simulink model "Cardiovascular"  (Simulink 6.4)
settings: Solver=ode45  StartTime=0.0  StopTime=50  MaxStep=0.01  MinStep=0.0000000000001  RelTol=1e-1
values from neighbouring files (symbols this model uses):
  A = 20.9    [Gas_Exchange_IC.m]    (also in getPneumonia.m = (LF1-LF2)/(1-exp(Rresolve*(t2(end)-t2(1)))))
  B = 92.8    [Gas_Exchange_IC.m]    (also in getPneumonia.m = LungFunction(end)-A)
  C = 10570    [Gas_Exchange_IC.m]
  D = -5.251    [Gas_Exchange_IC.m]
  fcs_max = 47.78    [Cardiovascular_IC.m]    (also in Reflex_Ursino_IC.m)
  fcs_min = 2.52    [Cardiovascular_IC.m]    (also in Reflex_Ursino_IC.m)
  ftbs_min = 0.1    [Cardiovascular_IC.m]    (also in SA_Node_Ursino_IC.m)
  HP_basal = 0.58    [Cardiovascular_IC.m]    (also in SA_Node_Ursino_IC.m)
  k_cs = 11.758    [Cardiovascular_IC.m]    (also in Reflex_Ursino_IC.m)
  Pn = 90    [Cardiovascular_IC.m]    (also in Reflex_Ursino_IC.m)
undefined symbols (not defined in the file or in its folder): Cbp, Cbv, Cep, Cev, Chp, Chv, Cla, Cmp, Cmv, Cpa, Cpp, Cpv, Cra, Csa, Csp, Csv, CvbO2_n, CvhO2_n, CvmO2_n, Dx, ftas_min, Gas_sleep, GbO2, Gbs_sleep, GhO2, GmO2, Gpara_sleep, initx, k_cs_sleep, KElv, KErv, KhCO2, KmCO2, Kr_vc, KRlv, KRrv, ksys, Lpa, Lsa, Mb, Mhn, Mm, P0lv, P0rv, PaCO2_n, Pn_sleep, R_vc_0, Rbpn, Rbv, Rev, Rhpn, Rhv, Rla, Rmv, Rpa, Rpp, Rpv, Rra, Rsa, Rsv ... (+25)
(part 1 of 2)
settings Model: LastModifiedBy=cPhonix
settings SolverCC: InitialStep=0.0000000000001
settings DataIOCC: SignalLoggingName=sigsOut
settings OptimizationCC: BooleanDataType=off
settings DebuggingCC: SolverPrmCheckMsg=none  StrictBusMsg=None
settings HardwareCC: TargetUnknown=on

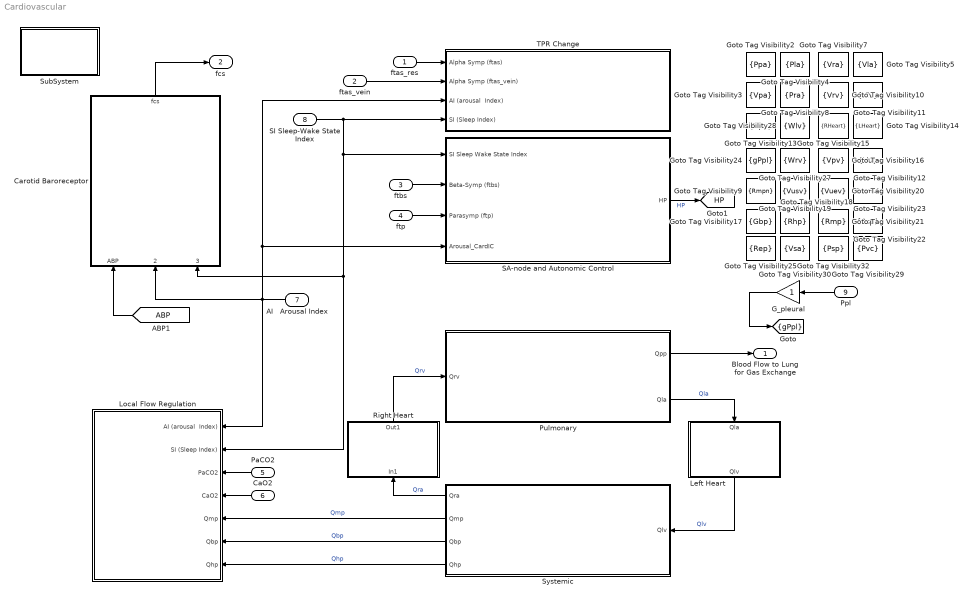
== system Cardiovascular ==
  ftas_res : Inport
  ftas_vein : Inport  Port=2
  ftbs : Inport  Port=3
  ftp : Inport  Port=4
  PaCO2 : Inport  Orientation=left  Port=5
  CaO2 : Inport  Orientation=left  Port=6
  AI   Arousal Index : Inport  Orientation=left  Port=7  DataType=double
  SI Sleep-Wake State Index : Inport  Port=8
  Ppl : Inport  Orientation=left  Port=9
  Carotid Baroreceptor : Subsystem  Orientation=up
      mask Display: disp('Carotid\n Baroreceptor')
  G_pleural : Gain  Orientation=left  SaturateOnIntegerOverflow=on
  Goto Tag Visibility10 : GotoTagVisibility  GotoTag=Vrv
  Goto Tag Visibility11 : GotoTagVisibility  GotoTag=Vlv
  Goto Tag Visibility12 : GotoTagVisibility  GotoTag=Vu
  Goto Tag Visibility13 : GotoTagVisibility  GotoTag=Vpp
  Goto Tag Visibility14 : GotoTagVisibility  GotoTag=LHeart
  Goto Tag Visibility15 : GotoTagVisibility  GotoTag=RHeart
  Goto Tag Visibility16 : GotoTagVisibility  GotoTag=Vpv
  Goto Tag Visibility17 : GotoTagVisibility  GotoTag=Gbp
  Goto Tag Visibility18 : GotoTagVisibility  GotoTag=Rhp
  Goto Tag Visibility19 : GotoTagVisibility  GotoTag=Vusv
  Goto Tag Visibility2 : GotoTagVisibility  GotoTag=Ppa
  Goto Tag Visibility20 : GotoTagVisibility  GotoTag=Vuev
  Goto Tag Visibility21 : GotoTagVisibility  GotoTag=Rmp
  Goto Tag Visibility22 : GotoTagVisibility  GotoTag=Rsp
  Goto Tag Visibility23 : GotoTagVisibility  GotoTag=Vumv
  Goto Tag Visibility24 : GotoTagVisibility  GotoTag=gPpl
  Goto Tag Visibility25 : GotoTagVisibility  GotoTag=Rep
  Goto Tag Visibility27 : GotoTagVisibility  GotoTag=Wrv
  Goto Tag Visibility28 : GotoTagVisibility  GotoTag=Wlv
  Goto Tag Visibility29 : GotoTagVisibility  GotoTag=Pvc
  Goto Tag Visibility3 : GotoTagVisibility  GotoTag=Vpa
  Goto Tag Visibility30 : GotoTagVisibility  GotoTag=Vsa
  Goto Tag Visibility32 : GotoTagVisibility  GotoTag=Psp
  Goto Tag Visibility4 : GotoTagVisibility  GotoTag=Pla
  Goto Tag Visibility5 : GotoTagVisibility  GotoTag=Vla
  Goto Tag Visibility7 : GotoTagVisibility  GotoTag=Vra
  Goto Tag Visibility8 : GotoTagVisibility  GotoTag=Pra
  Goto Tag Visibility9 : GotoTagVisibility  GotoTag=Rmpn
  Left Heart : Subsystem  Orientation=down
      mask Display: disp('LEFT HEART')
  Local Flow Regulation : Subsystem  Orientation=left
      mask Display: disp('Local Flow Regulation')
  Pulmonary : Subsystem
      mask Display: disp('PULMONARY CIRCULATORY SYSTEM')
  Right Heart : Subsystem  Orientation=up
      mask Display: disp('RIGHT HEART')
  SA-node and Autonomic Control : Subsystem
  SubSystem : Subsystem
      settings: OpenFcn=pneuma_variables
      mask Display: disp('"double click here"\n to load \nCardiovascular \ninitial values');
  Systemic : Subsystem  Orientation=left
      mask Display: disp('SYSTEMIC CIRULATORY SYSTEM')
  TPR Change : Subsystem
  Blood Flow to Lung for Gas Exchange : Outport
  fcs : Outport  Port=2
  tag scope: HP=global, gPpl=scoped
  wires:
  ftp/1 -> SA-node and Autonomic Control/3(Parasymp (ftp))
  ftbs/1 -> SA-node and Autonomic Control/2(Beta-Symp (ftbs))
  ftas_res/1 -> TPR Change/1(Alpha Symp (ftas))
  Carotid Baroreceptor/1(fcs) -> fcs/1
  SI Sleep-Wake State Index/1 -> SA-node and Autonomic Control/1(SI Sleep Wake State Index), Carotid Baroreceptor/3(SI Sleep Wake State Index), Local Flow Regulation/2("SI (Sleep Index) "), TPR Change/4("SI (Sleep Index) ")
  Ppl/1 -> G_pleural/1
  G_pleural/1 -> [gPpl]
  SA-node and Autonomic Control/1(HP) -> [HP]  "HP"
  [ABP] -> Carotid Baroreceptor/1(ABP)
  Systemic/1(Qra) -> Right Heart/1(In1)  "Qra"
  Left Heart/1(Qlv) -> Systemic/1(Qlv)  "Qlv"
  Right Heart/1(Out1) -> Pulmonary/1(Qrv)  "Qrv"
  Pulmonary/2(Qla) -> Left Heart/1(Qla)  "Qla"
  ftas_vein/1 -> TPR Change/2(Alpha Symp (ftas_vein))
  PaCO2/1 -> Local Flow Regulation/3(PaCO2)
  CaO2/1 -> Local Flow Regulation/4(CaO2)
  Systemic/2(Qmp) -> Local Flow Regulation/5(Qmp)  "Qmp"
  Systemic/3(Qbp) -> Local Flow Regulation/6(Qbp)  "Qbp"
  Systemic/4(Qhp) -> Local Flow Regulation/7(Qhp)  "Qhp"
  Pulmonary/1(Qpp) -> Blood Flow to Lung for Gas Exchange/1
  AI   Arousal Index/1 -> Carotid Baroreceptor/2("AI - Arousal Index "), SA-node and Autonomic Control/4(Arousal_CardIC), TPR Change/3(AI (arousal  Index)), Local Flow Regulation/1(AI (arousal  Index))

== system Cardiovascular/Carotid Baroreceptor ==
  ABP : Inport
  "AI - Arousal Index " : Inport  Port=2
  SI Sleep Wake State Index : Inport  Port=3
  Fcn : Fcn  Expr="(exp((u(1) - Pn + (1-u(2)) * u(3) * Pn_sleep ) / (  (1-u(2)) * u(3) *k_cs_sleep + k_cs) ) * fcs_max + fcs_min)/(exp((u(1) - Pn + (1-u(2)) * u(3) * Pn_sleep ) / (  (1-u(2)) * u(3) *k_cs_sleep + k_cs) ) +1) *1"
  Mux : Mux  Inputs=3
  Transfer Fcn : TransferFcn  Numerator=[touz 1]  Denominator=[toup 1]
  fcs : Outport
  wires:
  Fcn/1 -> fcs/1
  Mux/1 -> Fcn/1
  ABP/1 -> Transfer Fcn/1
  "AI - Arousal Index "/1 -> Mux/2
  SI Sleep Wake State Index/1 -> Mux/3
  Transfer Fcn/1 -> Mux/1

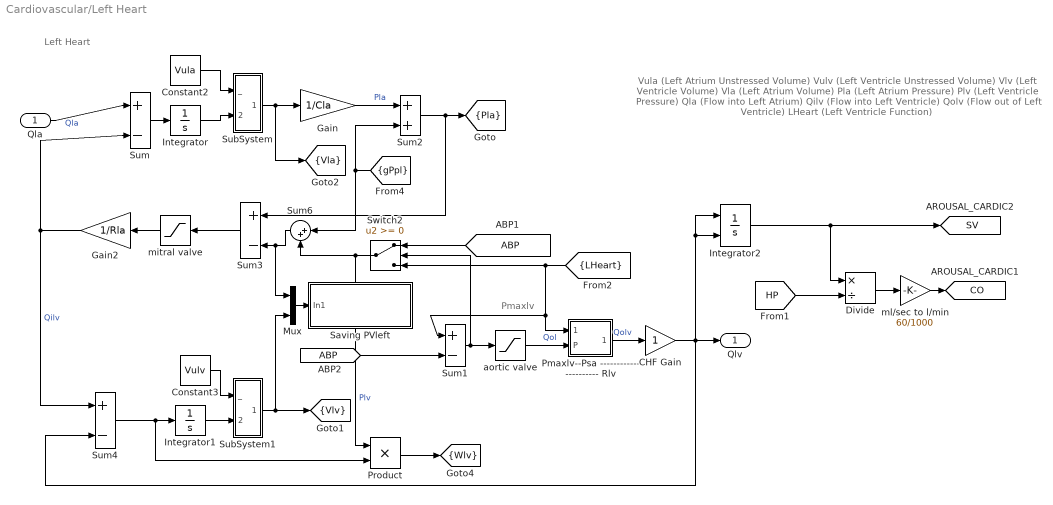
== system Cardiovascular/Left Heart ==
  note: Left Heart
  note: Vula (Left Atrium Unstressed Volume)
      | Vulv (Left Ventricle Unstressed Volume)
      | Vlv (Left Ventricle Volume)
      | Vla (Left Atrium Volume)
      | Pla (Left Atrium Pressure)
      | Plv (Left Ventricle Pressure)
      | Qla (Flow into Left Atrium)
      | Qilv (Flow into Left Ventricle)
      | Qolv (Flow out of Left Ventricle)
      | LHeart (Left Ventricle Function)
  note: Pmaxlv
  Qla : Inport
  CHF Gain : Gain
  Constant2 : Constant  Value=Vula  OutDataType=sfix(16)  ConRadixGroup=Use specified scaling  OutScaling=2^0  SampleTime=inf  FramePeriod=inf
  Constant3 : Constant  Value=Vulv  OutDataType=sfix(16)  ConRadixGroup=Use specified scaling  OutScaling=2^0  SampleTime=inf  FramePeriod=inf
  Divide : Product  Inputs=*/  OutScaling=2^-10
  Gain : Gain  Gain=1/Cla  SaturateOnIntegerOverflow=on
  Gain2 : Gain  Orientation=left  Gain=1/Rla  SaturateOnIntegerOverflow=on
  Integrator : Integrator
  Integrator1 : Integrator
  Integrator2 : Integrator  ExternalReset=rising
  Mux : Mux  Inputs=2
  Pmaxlv--Psa ---------------------- Rlv : Subsystem
  Product : Product  RndMeth=Zero
  Saving PVleft : Subsystem
  SubSystem : Subsystem
  SubSystem1 : Subsystem
  Sum : Sum  Inputs=|+-  SaturateOnIntegerOverflow=on  InputSameDT=on
  Sum1 : Sum  Inputs=+-  SaturateOnIntegerOverflow=on  InputSameDT=on
  Sum2 : Sum  SaturateOnIntegerOverflow=on  InputSameDT=on
  Sum3 : Sum  Orientation=left  Inputs=+-  SaturateOnIntegerOverflow=on  InputSameDT=on
  Sum4 : Sum  Inputs=+-  SaturateOnIntegerOverflow=on  InputSameDT=on
  Sum6 : Sum  Orientation=left  Inputs=|++
  Switch2 : Switch  Orientation=left  SaturateOnIntegerOverflow=on  InputSameDT=on
  aortic valve : Saturate  UpperLimit=inf  LowerLimit=0
  mitral valve : Saturate  Orientation=left  UpperLimit=inf  LowerLimit=0
  ml/sec to l/min : Gain  Gain=60/1000
  Qlv : Outport
  tag scope: CO=global, Pla=scoped, SV=global, Vla=scoped, Vlv=scoped, Wlv=scoped
  wires:
  Qla/1 -> Sum/1  "Qla"
  Sum/1 -> Integrator/1
  [ABP] -> Sum1/2
  Sum4/1 -> Integrator1/1, Product/2
  Gain2/1 -> Sum/2, Sum4/1  "Qilv"
  Pmaxlv--Psa ---------------------- Rlv/1(Flow) -> CHF Gain/1  "Qolv"
  Constant2/1 -> SubSystem/1(_)
  Constant3/1 -> SubSystem1/1(_)
  SubSystem/1(Out) -> Gain/1, [Vla]
  Sum1/1 -> aortic valve/1, Switch2/2
  [ABP] -> Switch2/1
  mitral valve/1 -> Gain2/1
  [LHeart] -> Switch2/3, Pmaxlv--Psa ---------------------- Rlv/1(Pmax), Sum1/1
  aortic valve/1 -> Pmaxlv--Psa ---------------------- Rlv/2(P)  "Qol"
  SubSystem1/1(Out) -> Mux/2, [Vlv]
  Integrator1/1 -> SubSystem1/2(+)
  Sum3/1 -> mitral valve/1
  Integrator/1 -> SubSystem/2(+)
  Gain/1 -> Sum2/1  "Pla"
  Sum2/1 -> [Pla], Sum3/1
  Switch2/1 -> Sum6/2, Product/1  "Plv"
  Sum6/1 -> Sum3/2, Mux/1
  [gPpl] -> Sum2/2, Sum6/1
  Product/1 -> [Wlv]
  CHF Gain/1 -> Qlv/1, Integrator2/2, Integrator2/1, Sum4/2
  Divide/1 -> ml/sec to l/min/1
  [HP] -> Divide/2
  Integrator2/1 -> Divide/1, [SV]
  ml/sec to l/min/1 -> [CO]
  Mux/1 -> Saving PVleft/1(In1)

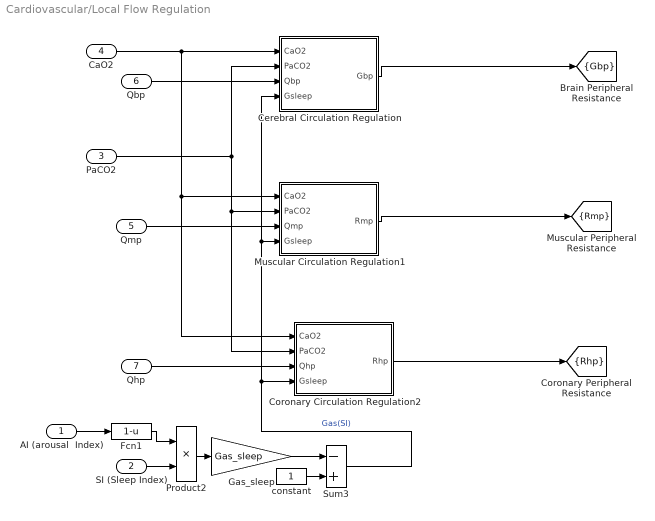
== system Cardiovascular/Local Flow Regulation ==
  AI (arousal  Index) : Inport
  "SI (Sleep Index) " : Inport  Port=2
  PaCO2 : Inport  Port=3
  CaO2 : Inport  Port=4
  Qmp : Inport  Port=5
  Qbp : Inport  Port=6
  Qhp : Inport  Port=7
  Cerebral Circulation Regulation : Subsystem
  Coronary Circulation Regulation2 : Subsystem
  Fcn1 : Fcn  Expr=1-u
  Gas_sleep : Gain  Gain=Gas_sleep  SaturateOnIntegerOverflow=on
  Muscular Circulation Regulation1 : Subsystem
  Product2 : Product  SaturateOnIntegerOverflow=on  InputSameDT=on
  Sum3 : Sum  Inputs=-+  SaturateOnIntegerOverflow=on  InputSameDT=on
  constant : Constant  Value=1  OutDataType=sfix(16)  ConRadixGroup=Use specified scaling  OutScaling=2^0  SampleTime=inf  FramePeriod=inf
  tag scope: Gbp=scoped, Rhp=scoped, Rmp=scoped
  wires:
  CaO2/1 -> Cerebral Circulation Regulation/1(CaO2), Muscular Circulation Regulation1/1(CaO2), Coronary Circulation Regulation2/1(CaO2)
  PaCO2/1 -> Cerebral Circulation Regulation/2(PaCO2), Muscular Circulation Regulation1/2(PaCO2), Coronary Circulation Regulation2/2(PaCO2)
  Cerebral Circulation Regulation/1(Gbp) -> [Gbp]
  Muscular Circulation Regulation1/1(Rmp) -> [Rmp]
  Coronary Circulation Regulation2/1(Rhp) -> [Rhp]
  Qbp/1 -> Cerebral Circulation Regulation/3(Qbp)
  Qmp/1 -> Muscular Circulation Regulation1/3(Qmp)
  Qhp/1 -> Coronary Circulation Regulation2/3(Qhp)
  AI (arousal  Index)/1 -> Fcn1/1
  "SI (Sleep Index) "/1 -> Product2/2
  Fcn1/1 -> Product2/1
  Product2/1 -> Gas_sleep/1
  constant/1 -> Sum3/2
  Gas_sleep/1 -> Sum3/1
  Sum3/1 -> Coronary Circulation Regulation2/4(Gsleep), Muscular Circulation Regulation1/4(Gsleep), Cerebral Circulation Regulation/4(Gsleep)  "Gas(SI)"

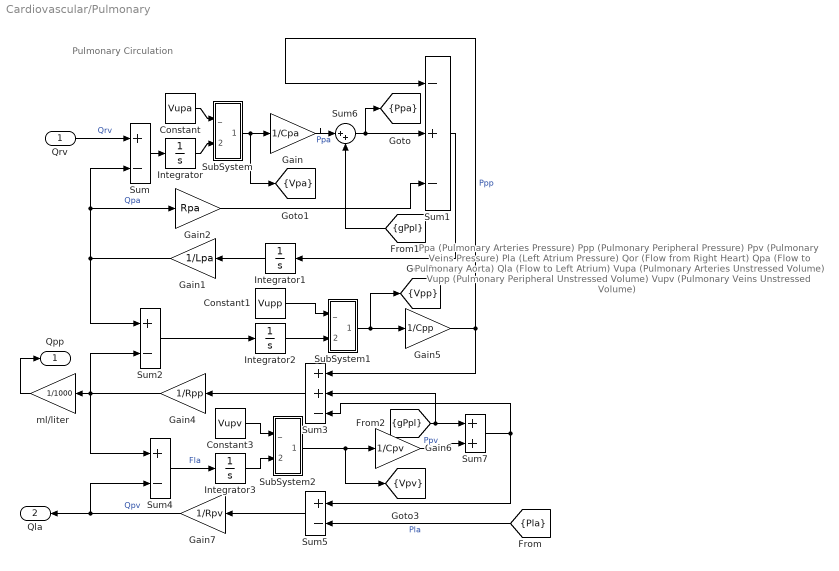
== system Cardiovascular/Pulmonary ==
  note: Ppa (Pulmonary Arteries Pressure)
      | Ppp (Pulmonary Peripheral Pressure)
      | Ppv (Pulmonary Veins Pressure)
      | Pla (Left Atrium Pressure)
      | Qor (Flow from Right Heart)
      | Qpa (Flow to Pulmonary Aorta)
      | Qla (Flow to Left Atrium)
      | Vupa (Pulmonary Arteries Unstressed Volume)
      | Vupp (Pulmonary Peripheral Unstressed Volume)
      | Vupv (Pulmonary Veins Unstressed Volume)
  note: Pulmonary Circulation
  Qrv : Inport
  Constant : Constant  Value=Vupa  OutDataType=sfix(16)  ConRadixGroup=Use specified scaling  OutScaling=2^0  SampleTime=inf  FramePeriod=inf
  Constant1 : Constant  Value=Vupp  OutDataType=sfix(16)  ConRadixGroup=Use specified scaling  OutScaling=2^0  SampleTime=inf  FramePeriod=inf
  Constant3 : Constant  Value=Vupv  OutDataType=sfix(16)  ConRadixGroup=Use specified scaling  OutScaling=2^0  SampleTime=inf  FramePeriod=inf
  Gain : Gain  Gain=1/Cpa  SaturateOnIntegerOverflow=on
  Gain1 : Gain  Orientation=left  Gain=1/Lpa  SaturateOnIntegerOverflow=on
  Gain2 : Gain  Gain=Rpa  SaturateOnIntegerOverflow=on
  Gain4 : Gain  Orientation=left  Gain=1/Rpp  SaturateOnIntegerOverflow=on
  Gain5 : Gain  Gain=1/Cpp  SaturateOnIntegerOverflow=on
  Gain6 : Gain  Gain=1/Cpv  SaturateOnIntegerOverflow=on
  Gain7 : Gain  Orientation=left  Gain=1/Rpv  SaturateOnIntegerOverflow=on
  Integrator : Integrator  InitialCondition=100
  Integrator1 : Integrator  Orientation=left
  Integrator2 : Integrator  InitialCondition=100
  Integrator3 : Integrator
  SubSystem : Subsystem
  SubSystem1 : Subsystem
  SubSystem2 : Subsystem
  Sum : Sum  Inputs=+-  SaturateOnIntegerOverflow=on  InputSameDT=on
  Sum1 : Sum  Inputs=-+-  SaturateOnIntegerOverflow=on  InputSameDT=on
  Sum2 : Sum  Inputs=+-  SaturateOnIntegerOverflow=on  InputSameDT=on
  Sum3 : Sum  Orientation=left  Inputs=++-  SaturateOnIntegerOverflow=on  InputSameDT=on
  Sum4 : Sum  Inputs=+-  SaturateOnIntegerOverflow=on  InputSameDT=on
  Sum5 : Sum  Orientation=left  Inputs=+-  SaturateOnIntegerOverflow=on  InputSameDT=on
  Sum6 : Sum  Inputs=|++
  Sum7 : Sum
  ml/liter : Gain  Orientation=left  Gain=1/1000  SaturateOnIntegerOverflow=on
  Qpp : Outport
  Qla : Outport  Orientation=left  Port=2
  tag scope: Ppa=scoped, Vpa=scoped, Vpp=scoped, Vpv=scoped
  wires:
  Qrv/1 -> Sum/1  "Qrv"
  Sum/1 -> Integrator/1
  Integrator1/1 -> Gain1/1
  Sum1/1 -> Integrator1/1
  Gain2/1 -> Sum1/3
  Gain1/1 -> Sum/2, Gain2/1, Sum2/1  "Qpa"
  Sum2/1 -> Integrator2/1
  Gain5/1 -> Sum1/1, Sum3/1  "Ppp"
  Sum3/1 -> Gain4/1
  Gain4/1 -> Sum2/2, Sum4/1, ml/liter/1
  Sum5/1 -> Gain7/1
  [Pla] -> Sum5/2  "Pla"
  Sum4/1 -> Integrator3/1  "Fla"
  SubSystem/1(Out) -> Gain/1, [Vpa]
  SubSystem1/1(Out) -> Gain5/1, [Vpp]
  SubSystem2/1(Out) -> Gain6/1, [Vpv]
  Integrator/1 -> SubSystem/2(+)
  Constant/1 -> SubSystem/1(_)
  Constant1/1 -> SubSystem1/1(_)
  Integrator2/1 -> SubSystem1/2(+)
  Integrator3/1 -> SubSystem2/2(+)
  Gain7/1 -> Qla/1, Sum4/2  "Qpv"
  Constant3/1 -> SubSystem2/1(_)
  Gain/1 -> Sum6/1  "Ppa"
  Sum6/1 -> Sum1/2, [Ppa]
  Gain6/1 -> Sum7/2  "Ppv"
  Sum7/1 -> Sum5/1, Sum3/3
  [gPpl] -> Sum7/1, Sum3/2
  ml/liter/1 -> Qpp/1
  [gPpl] -> Sum6/2

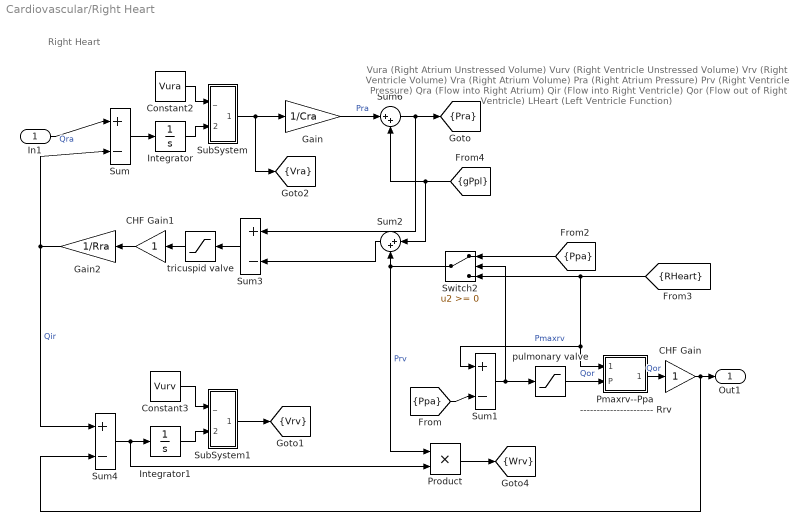
== system Cardiovascular/Right Heart ==
  note: Right Heart
  note: Vura (Right Atrium Unstressed Volume)
      | Vurv (Right Ventricle Unstressed Volume)
      | Vrv (Right Ventricle Volume)
      | Vra (Right Atrium Volume)
      | Pra (Right Atrium Pressure)
      | Prv (Right Ventricle Pressure)
      | Qra (Flow into Right Atrium)
      | Qir (Flow into Right Ventricle)
      | Qor (Flow out of Right Ventricle)
      | LHeart (Left Ventricle Function)
  In1 : Inport
  CHF Gain : Gain
  CHF Gain1 : Gain  Orientation=left
  Constant2 : Constant  Value=Vura  OutDataType=sfix(16)  ConRadixGroup=Use specified scaling  OutScaling=2^0  SampleTime=inf  FramePeriod=inf
  Constant3 : Constant  Value=Vurv  OutDataType=sfix(16)  ConRadixGroup=Use specified scaling  OutScaling=2^0  SampleTime=inf  FramePeriod=inf
  Gain : Gain  Gain=1/Cra  SaturateOnIntegerOverflow=on
  Gain2 : Gain  Orientation=left  Gain=1/Rra  SaturateOnIntegerOverflow=on
  Integrator : Integrator
  Integrator1 : Integrator
  Pmaxrv--Ppa ---------------------- Rrv : Subsystem
  Product : Product  RndMeth=Zero
  SubSystem : Subsystem
  SubSystem1 : Subsystem
  Sum : Sum  Inputs=|+-  SaturateOnIntegerOverflow=on  InputSameDT=on
  Sum1 : Sum  Inputs=|+-  SaturateOnIntegerOverflow=on  InputSameDT=on
  Sum2 : Sum  Orientation=left  Inputs=|++
  Sum3 : Sum  Orientation=left  Inputs=+-  SaturateOnIntegerOverflow=on  InputSameDT=on
  Sum4 : Sum  Inputs=+-  SaturateOnIntegerOverflow=on  InputSameDT=on
  Sum6 : Sum  Inputs=|++
  Switch2 : Switch  Orientation=left  SaturateOnIntegerOverflow=on  InputSameDT=on
  pulmonary valve : Saturate  UpperLimit=inf  LowerLimit=0
  tricuspid valve : Saturate  Orientation=left  UpperLimit=inf  LowerLimit=0
  Out1 : Outport
  tag scope: Pra=scoped, Vra=scoped, Vrv=scoped, Wrv=scoped
  wires:
  In1/1 -> Sum/1  "Qra"
  Sum/1 -> Integrator/1
  [Ppa] -> Sum1/2
  Gain2/1 -> Sum/2, Sum4/1  "Qir"
  Integrator/1 -> SubSystem/2(+)
  Constant2/1 -> SubSystem/1(_)
  SubSystem1/1(Out) -> [Vrv]
  SubSystem/1(Out) -> Gain/1, [Vra]
  Constant3/1 -> SubSystem1/1(_)
  Integrator1/1 -> SubSystem1/2(+)
  Sum1/1 -> pulmonary valve/1, Switch2/2
  [Ppa] -> Switch2/1
  tricuspid valve/1 -> CHF Gain1/1
  pulmonary valve/1 -> Pmaxrv--Ppa ---------------------- Rrv/2(P)  "Qor"
  Pmaxrv--Ppa ---------------------- Rrv/1(Flow) -> CHF Gain/1  "Qor"
  [RHeart] -> Switch2/3, Pmaxrv--Ppa ---------------------- Rrv/1(Pmax), Sum1/1  "Pmaxrv"
  Sum4/1 -> Integrator1/1, Product/2
  Sum3/1 -> tricuspid valve/1
  Gain/1 -> Sum6/1  "Pra"
  Sum6/1 -> [Pra], Sum3/1
  Switch2/1 -> Sum2/2, Product/1  "Prv"
  Sum2/1 -> Sum3/2
  [gPpl] -> Sum2/1, Sum6/2
  Product/1 -> [Wrv]
  CHF Gain/1 -> Out1/1, Sum4/2
  CHF Gain1/1 -> Gain2/1

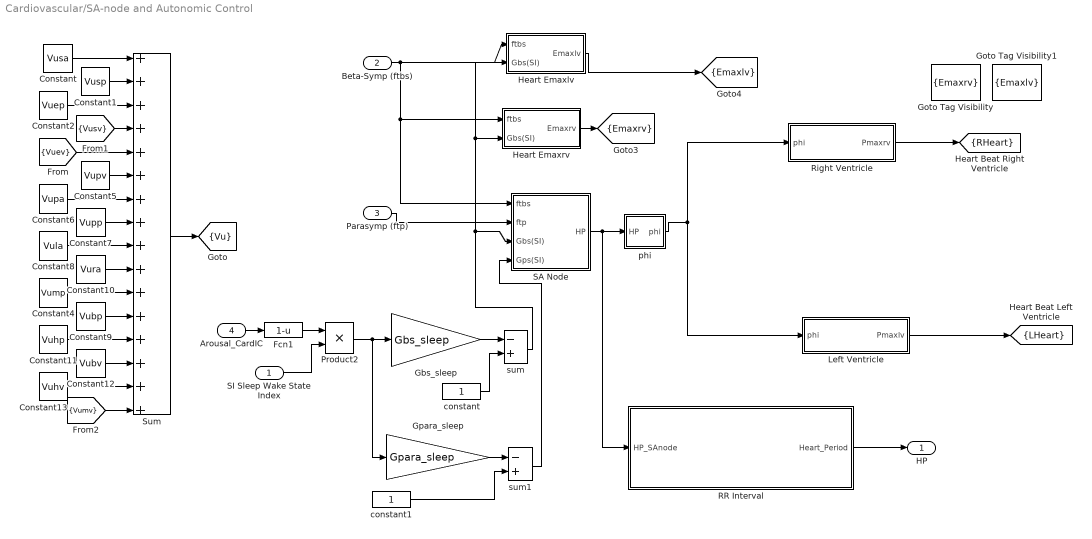
== system Cardiovascular/SA-node and Autonomic Control ==
  SI Sleep Wake State Index : Inport
  Beta-Symp (ftbs) : Inport  Port=2
  Parasymp (ftp) : Inport  Port=3
  Arousal_CardIC : Inport  Port=4
  Constant : Constant  Value=Vusa  OutDataType=sfix(16)  ConRadixGroup=Use specified scaling  OutScaling=2^0  SampleTime=inf  FramePeriod=inf
  Constant1 : Constant  Value=Vusp  OutDataType=sfix(16)  ConRadixGroup=Use specified scaling  OutScaling=2^0  SampleTime=inf  FramePeriod=inf
  Constant10 : Constant  Value=Vura  OutDataType=sfix(16)  ConRadixGroup=Use specified scaling  OutScaling=2^0  SampleTime=inf  FramePeriod=inf
  Constant11 : Constant  Value=Vuhp  OutDataType=sfix(16)  ConRadixGroup=Use specified scaling  OutScaling=2^0  SampleTime=inf  FramePeriod=inf
  Constant12 : Constant  Value=Vubv  OutDataType=sfix(16)  ConRadixGroup=Use specified scaling  OutScaling=2^0  SampleTime=inf  FramePeriod=inf
  Constant13 : Constant  Value=Vuhv  OutDataType=sfix(16)  ConRadixGroup=Use specified scaling  OutScaling=2^0  SampleTime=inf  FramePeriod=inf
  Constant2 : Constant  Value=Vuep  OutDataType=sfix(16)  ConRadixGroup=Use specified scaling  OutScaling=2^0  SampleTime=inf  FramePeriod=inf
  Constant4 : Constant  Value=Vump  OutDataType=sfix(16)  ConRadixGroup=Use specified scaling  OutScaling=2^0  SampleTime=inf  FramePeriod=inf
  Constant5 : Constant  Value=Vupv  OutDataType=sfix(16)  ConRadixGroup=Use specified scaling  OutScaling=2^0  SampleTime=inf  FramePeriod=inf
  Constant6 : Constant  Value=Vupa  OutDataType=sfix(16)  ConRadixGroup=Use specified scaling  OutScaling=2^0  SampleTime=inf  FramePeriod=inf
  Constant7 : Constant  Value=Vupp  OutDataType=sfix(16)  ConRadixGroup=Use specified scaling  OutScaling=2^0  SampleTime=inf  FramePeriod=inf
  Constant8 : Constant  Value=Vula  OutDataType=sfix(16)  ConRadixGroup=Use specified scaling  OutScaling=2^0  SampleTime=inf  FramePeriod=inf
  Constant9 : Constant  Value=Vubp  OutDataType=sfix(16)  ConRadixGroup=Use specified scaling  OutScaling=2^0  SampleTime=inf  FramePeriod=inf
  Fcn1 : Fcn  Expr=1-u
  Gbs_sleep : Gain  Gain=Gbs_sleep  SaturateOnIntegerOverflow=on
  Goto Tag Visibility : GotoTagVisibility  GotoTag=Emaxrv
  Goto Tag Visibility1 : GotoTagVisibility  GotoTag=Emaxlv
  Gpara_sleep : Gain  Gain=Gpara_sleep  SaturateOnIntegerOverflow=on
  Heart Emaxlv : Subsystem
  Heart Emaxrv : Subsystem
  Left Ventricle : Subsystem
  Product2 : Product  SaturateOnIntegerOverflow=on  InputSameDT=on
  RR Interval : Subsystem
  Right Ventricle : Subsystem
  SA Node : Subsystem
  Sum : Sum  Inputs=++++++++++++++++  SaturateOnIntegerOverflow=on  InputSameDT=on
  constant : Constant  Value=1  OutDataType=sfix(16)  ConRadixGroup=Use specified scaling  OutScaling=2^0  SampleTime=inf  FramePeriod=inf
  constant1 : Constant  Value=1  OutDataType=sfix(16)  ConRadixGroup=Use specified scaling  OutScaling=2^0  SampleTime=inf  FramePeriod=inf
  phi : Subsystem
  sum : Sum  Inputs=-+  SaturateOnIntegerOverflow=on  InputSameDT=on
  sum1 : Sum  Inputs=-+  SaturateOnIntegerOverflow=on  InputSameDT=on
  HP : Outport
  tag scope: Emaxlv=scoped, Emaxrv=scoped, LHeart=scoped, RHeart=scoped, Vu=scoped
  wires:
  Arousal_CardIC/1 -> Fcn1/1
  SI Sleep Wake State Index/1 -> Product2/2
  sum/1 -> Heart Emaxrv/2(Gbs(SI)), Heart Emaxlv/2(Gbs(SI)), SA Node/3(Gbs(SI))
  sum1/1 -> SA Node/4(Gps(SI))
  Fcn1/1 -> Product2/1
  Product2/1 -> Gbs_sleep/1, Gpara_sleep/1
  Gbs_sleep/1 -> sum/1
  constant/1 -> sum/2
  Gpara_sleep/1 -> sum1/1
  constant1/1 -> sum1/2
  Sum/1 -> [Vu]
  Constant/1 -> Sum/1
  Constant2/1 -> Sum/3
  Constant1/1 -> Sum/2
  [Vusv] -> Sum/4
  [Vuev] -> Sum/5
  Constant5/1 -> Sum/6
  Constant6/1 -> Sum/7
  Constant7/1 -> Sum/8
  Constant8/1 -> Sum/9
  Constant10/1 -> Sum/10
  Constant4/1 -> Sum/11
  Constant9/1 -> Sum/12
  Constant11/1 -> Sum/13
  Constant12/1 -> Sum/14
  Constant13/1 -> Sum/15
  [Vumv] -> Sum/16
  phi/1(phi) -> Right Ventricle/1(phi), Left Ventricle/1(phi)
  Right Ventricle/1(Pmaxrv) -> [RHeart]
  Left Ventricle/1(Pmaxlv) -> [LHeart]
  SA Node/1(HP) -> phi/1(HP), RR Interval/1(HP_SAnode)
  Heart Emaxrv/1(Emaxrv) -> [Emaxrv]
  Heart Emaxlv/1(Emaxlv) -> [Emaxlv]
  Beta-Symp (ftbs)/1 -> Heart Emaxrv/1(ftbs), SA Node/1(ftbs), Heart Emaxlv/1(ftbs)
  Parasymp (ftp)/1 -> SA Node/2(ftp)
  RR Interval/1(Heart_Period) -> HP/1

== system Cardiovascular/SubSystem ==

== system Cardiovascular/Systemic ==
  note: Psa (Systemic Arteries Pressure)
      | Psp (Splanchnic Peripheral Pressure)
      | Pep (Extrasplanchnic Peripheral Pressure)
      | Psv (Splanchnic Venous Pressure)
      | Pvc (Vena Cava Pressure)
      | Pra (Right Atrium Pressure)
      | For (Flow from Left Heart)
      | Fsa (Flow to Systemic Aorta)
      | Fil (Flow to Left Atrium)
      | Fvc (Flow to Vena Cava)
      | Fra (Flow to Right Atrium)
      | Vusa (Systemic Arteries Unstressed Volume)
      | Vusp (Extrasplanchnic Venous Unstressed Volume)
      | Vuep (Splanchnic Venous Unstressed Volume)
      | Vuev (Extrasplanchnic Venous Unstressed Volume)
      | Vusv (Splanchnic Venous Unstressed Volume)
  note: Systemic Circulation
  Qlv : Inport
  Goto Tag Visibility7 : GotoTagVisibility  GotoTag=Vvc
  Systemic  Arteries : Subsystem
  Systemic  Peripheral & Venous Circulation : Subsystem
  Vena Cava : Subsystem
  Qra : Outport
  Qmp : Outport  Port=2
  Qbp : Outport  Port=3
  Qhp : Outport  Port=4
  wires:
  Qlv/1 -> Systemic  Arteries/1(Qlv)  "Fol"
  Systemic  Arteries/1(Qsa) -> Systemic  Peripheral & Venous Circulation/1(Qsa)
  Vena Cava/1(Qra) -> Qra/1
  Systemic  Peripheral & Venous Circulation/1(Qvc) -> Vena Cava/1(Qvc)
  Systemic  Peripheral & Venous Circulation/2(Qmp) -> Qmp/1
  Systemic  Peripheral & Venous Circulation/3(Qbp) -> Qbp/1
  Systemic  Peripheral & Venous Circulation/4(Qhp) -> Qhp/1

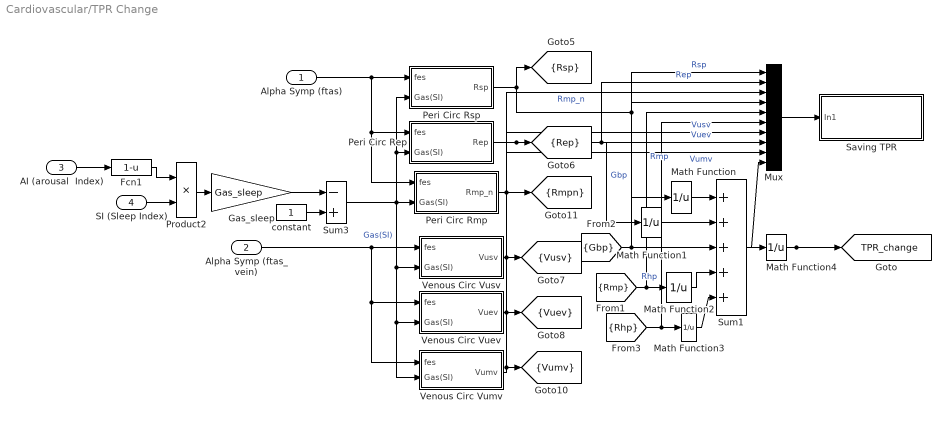
== system Cardiovascular/TPR Change ==
  Alpha Symp (ftas) : Inport
  Alpha Symp (ftas_vein) : Inport  Port=2
  AI (arousal  Index) : Inport  Port=3
  "SI (Sleep Index) " : Inport  Port=4
  Fcn1 : Fcn  Expr=1-u
  Gas_sleep : Gain  Gain=Gas_sleep  SaturateOnIntegerOverflow=on
  Math Function{,1..4} (5 alike) : Math  Operator=reciprocal  SaturateOnIntegerOverflow=on
  Mux : Mux  Inputs=10
  Peri Circ Rep : Subsystem
  Peri Circ Rmp : Subsystem
  Peri Circ Rsp : Subsystem
  Product2 : Product  SaturateOnIntegerOverflow=on  InputSameDT=on
  Saving TPR : Subsystem
  Sum1 : Sum  Inputs=+++++  SaturateOnIntegerOverflow=on  InputSameDT=on
  Sum3 : Sum  Inputs=-+  SaturateOnIntegerOverflow=on  InputSameDT=on
  Venous Circ Vuev : Subsystem
  Venous Circ Vumv : Subsystem
  Venous Circ Vusv : Subsystem
  constant : Constant  Value=1  OutDataType=sfix(16)  ConRadixGroup=Use specified scaling  OutScaling=2^0  SampleTime=inf  FramePeriod=inf
  tag scope: Rep=scoped, Rmpn=scoped, Rsp=scoped, TPR_change=global, Vuev=scoped, Vumv=scoped, Vusv=scoped
  wires:
  AI (arousal  Index)/1 -> Fcn1/1
  "SI (Sleep Index) "/1 -> Product2/2
  Fcn1/1 -> Product2/1
  Product2/1 -> Gas_sleep/1
  constant/1 -> Sum3/2
  Gas_sleep/1 -> Sum3/1
  Peri Circ Rep/1(Rep) -> [Rep], Math Function1/1, Mux/2  "Rep"
  Venous Circ Vusv/1(Vusv) -> [Vusv], Mux/7  "Vusv"
  Venous Circ Vuev/1(Vuev) -> [Vuev], Mux/8  "Vuev"
  Peri Circ Rsp/1(Rsp) -> [Rsp], Math Function/1, Mux/1  "Rsp"
  Venous Circ Vumv/1(Vumv) -> [Vumv], Mux/9  "Vumv"
  Peri Circ Rmp/1(Rmp_n) -> [Rmpn], Mux/3  "Rmp_n"
  Alpha Symp (ftas)/1 -> Peri Circ Rep/1(fes), Peri Circ Rmp/1(fes), Peri Circ Rsp/1(fes)
  Sum3/1 -> Peri Circ Rsp/2(Gas(SI)), Peri Circ Rep/2(Gas(SI)), Venous Circ Vusv/2(Gas(SI)), Venous Circ Vuev/2(Gas(SI)), Venous Circ Vumv/2(Gas(SI)), Peri Circ Rmp/2(Gas(SI))  "Gas(SI)"
  Alpha Symp (ftas_vein)/1 -> Venous Circ Vusv/1(fes), Venous Circ Vuev/1(fes), Venous Circ Vumv/1(fes)
  Sum1/1 -> Math Function4/1
  [Gbp] -> Sum1/3, Mux/4  "Gbp"
  [Rmp] -> Math Function2/1, Mux/5  "Rmp"
  [Rhp] -> Math Function3/1, Mux/6  "Rhp"
  Math Function/1 -> Sum1/1
  Math Function1/1 -> Sum1/2
  Math Function2/1 -> Sum1/4
  Math Function3/1 -> Sum1/5
  Math Function4/1 -> [TPR_change], Mux/10
  Mux/1 -> Saving TPR/1(In1)

== system Cardiovascular/Left Heart/Pmaxlv--Psa ---------------------- Rlv ==
  Pmax : Inport
  P : Inport  Port=2
  CHF Gain : Gain
  Gain : Gain  Gain=KRlv  SaturateOnIntegerOverflow=on
  Product : Product  Inputs=/*  SaturateOnIntegerOverflow=on  RndMeth=Zero  InputSameDT=on
  Saturation : Saturate  UpperLimit=inf  LowerLimit=0.01
  Flow : Outport
  wires:
  Pmax/1 -> CHF Gain/1
  Gain/1 -> Saturation/1
  P/1 -> Product/2
  Saturation/1 -> Product/1
  Product/1 -> Flow/1
  CHF Gain/1 -> Gain/1

== system Cardiovascular/Left Heart/Saving PVleft ==
  In1 : Inport
  Clock : Clock
      settings: Decimation=10
  Gain : Gain  Gain=1/(3600*24*7)
  Rounding Function : Rounding
  Switch Case : SwitchCase  CaseConditions={0,1,2,3,4,5,6,7,8}  SampleTime=0.1
  Switch Case Action Subsystem : Subsystem  TreatAsAtomicUnit=on
  Switch Case Action Subsystem1 : Subsystem  TreatAsAtomicUnit=on
  Switch Case Action Subsystem2 : Subsystem  TreatAsAtomicUnit=on
  Switch Case Action Subsystem3 : Subsystem  TreatAsAtomicUnit=on
  Switch Case Action Subsystem4 : Subsystem  TreatAsAtomicUnit=on
  Switch Case Action Subsystem5 : Subsystem  TreatAsAtomicUnit=on
  Switch Case Action Subsystem6 : Subsystem  TreatAsAtomicUnit=on
  Switch Case Action Subsystem7 : Subsystem  TreatAsAtomicUnit=on
  Switch Case Action Subsystem8 : Subsystem  TreatAsAtomicUnit=on
  Switch Case Action Subsystem9 : Subsystem  TreatAsAtomicUnit=on
  wires:
  Clock/1 -> Gain/1
  Switch Case/1 -> Switch Case Action Subsystem/Action
  Switch Case/2 -> Switch Case Action Subsystem1/Action
  Switch Case/3 -> Switch Case Action Subsystem2/Action
  Switch Case/10 -> Switch Case Action Subsystem3/Action
  Rounding Function/1 -> Switch Case/1
  In1/1 -> Switch Case Action Subsystem/1(In1), Switch Case Action Subsystem1/1(In1), Switch Case Action Subsystem2/1(In1), Switch Case Action Subsystem5/1(In1), Switch Case Action Subsystem3/1(In1), Switch Case Action Subsystem9/1(In1), Switch Case Action Subsystem8/1(In1), Switch Case Action Subsystem7/1(In1), Switch Case Action Subsystem6/1(In1), Switch Case Action Subsystem4/1(In1)
  Gain/1 -> Rounding Function/1
  Switch Case/4 -> Switch Case Action Subsystem4/Action
  Switch Case/5 -> Switch Case Action Subsystem5/Action
  Switch Case/6 -> Switch Case Action Subsystem6/Action
  Switch Case/7 -> Switch Case Action Subsystem7/Action
  Switch Case/8 -> Switch Case Action Subsystem8/Action
  Switch Case/9 -> Switch Case Action Subsystem9/Action

== system Cardiovascular/Left Heart/SubSystem ==
  _ : Inport
  + : Inport  Port=2
  Saturation : Saturate  UpperLimit=10000  LowerLimit=0
  Sum : Sum  Inputs=|-+  SaturateOnIntegerOverflow=on  InputSameDT=on
  Out : Outport
  wires:
  _/1 -> Sum/1
  +/1 -> Sum/2
  Sum/1 -> Saturation/1
  Saturation/1 -> Out/1

== system Cardiovascular/Left Heart/SubSystem1 ==
  _ : Inport
  + : Inport  Port=2
  Saturation : Saturate  UpperLimit=10000  LowerLimit=0
  Sum : Sum  Inputs=|-+  SaturateOnIntegerOverflow=on  InputSameDT=on
  Out : Outport
  wires:
  Saturation/1 -> Out/1
  Sum/1 -> Saturation/1
  +/1 -> Sum/2
  _/1 -> Sum/1

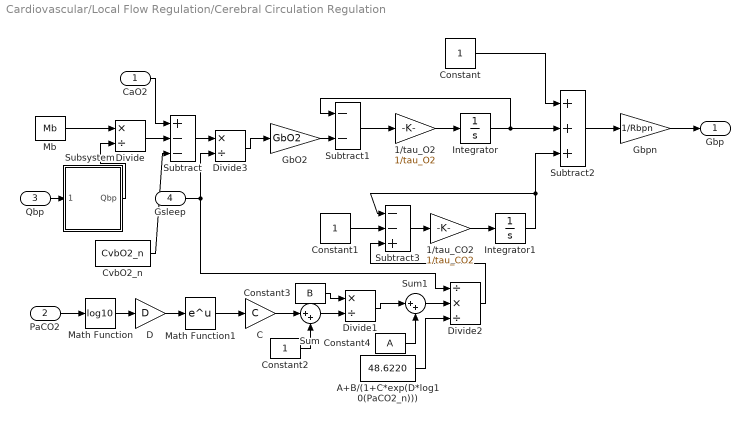
== system Cardiovascular/Local Flow Regulation/Cerebral Circulation Regulation ==
  CaO2 : Inport
  PaCO2 : Inport  Port=2
  Qbp : Inport  Port=3
  Gsleep : Inport  Port=4
  " A+B/(1+C*exp(D*log10(PaCO2_n)))" : Constant  Value=48.6220  OutDataType=sfix(16)  ConRadixGroup=Use specified scaling  OutScaling=2^0  SampleTime=inf  FramePeriod=inf
  1/tau_CO2 : Gain  Gain=1/tau_CO2
  1/tau_O2 : Gain  Gain=1/tau_O2
  C : Gain  Gain=C
  Constant : Constant  Value=1  OutDataType=sfix(16)  ConRadixGroup=Use specified scaling  OutScaling=2^0  SampleTime=inf  FramePeriod=inf
  Constant1 : Constant  Value=1  OutDataType=sfix(16)  ConRadixGroup=Use specified scaling  OutScaling=2^0  SampleTime=inf  FramePeriod=inf
  Constant2 : Constant  Value=1  OutDataType=sfix(16)  ConRadixGroup=Use specified scaling  OutScaling=2^0  SampleTime=inf  FramePeriod=inf
  Constant3 : Constant  Value=B  OutDataType=sfix(16)  ConRadixGroup=Use specified scaling  OutScaling=2^0  SampleTime=inf  FramePeriod=inf
  Constant4 : Constant  Value=A  OutDataType=sfix(16)  ConRadixGroup=Use specified scaling  OutScaling=2^0  SampleTime=inf  FramePeriod=inf
  CvbO2_n : Constant  Value=CvbO2_n  OutDataType=sfix(16)  ConRadixGroup=Use specified scaling  OutScaling=2^0  SampleTime=inf  FramePeriod=inf
  D : Gain  Gain=D
  Divide : Product  Inputs=*/  OutScaling=2^-10
  Divide1 : Product  Inputs=*/  OutScaling=2^-10
  Divide2 : Product  Inputs=/*/  OutScaling=2^-10
  Divide3 : Product  Inputs=*/  OutScaling=2^-10
  GbO2 : Gain  Gain=GbO2
  Gbpn : Gain  Gain=1/Rbpn
  Integrator : Integrator
  Integrator1 : Integrator
  Math Function : Math  Operator=log10  SaturateOnIntegerOverflow=on
  Math Function1 : Math  SaturateOnIntegerOverflow=on
  Mb : Constant  Value=Mb  OutDataType=sfix(16)  ConRadixGroup=Use specified scaling  OutScaling=2^0  SampleTime=inf  FramePeriod=inf
  Subsystem : Subsystem
  Subtract : Sum  Inputs=+--  OutScaling=2^-10
  Subtract1 : Sum  Inputs=--  OutScaling=2^-10
  Subtract2 : Sum  Inputs=+++  OutScaling=2^-10
  Subtract3 : Sum  Inputs=--+  OutScaling=2^-10
  Sum : Sum  Inputs=|++
  Sum1 : Sum  Inputs=|++
  Gbp : Outport
  wires:
  Mb/1 -> Divide/1
  Divide/1 -> Subtract/2
  CvbO2_n/1 -> Subtract/3
  Subtract/1 -> Divide3/1
  GbO2/1 -> Subtract1/2
  Subtract1/1 -> 1/tau_O2/1
  1/tau_O2/1 -> Integrator/1
  Integrator/1 -> Subtract1/1, Subtract2/2
  Constant/1 -> Subtract2/1
  1/tau_CO2/1 -> Integrator1/1
  Integrator1/1 -> Subtract2/3, Subtract3/1
  Subtract3/1 -> 1/tau_CO2/1
  Constant1/1 -> Subtract3/2
  Math Function/1 -> D/1
  D/1 -> Math Function1/1
  Math Function1/1 -> C/1
  C/1 -> Sum/1
  Constant2/1 -> Sum/2
  Constant3/1 -> Divide1/1
  Sum/1 -> Divide1/2
  Divide1/1 -> Sum1/1
  Constant4/1 -> Sum1/2
  Sum1/1 -> Divide2/2
  " A+B/(1+C*exp(D*log10(PaCO2_n)))"/1 -> Divide2/3
  Divide2/1 -> Subtract3/3
  Gbpn/1 -> Gbp/1
  CaO2/1 -> Subtract/1
  PaCO2/1 -> Math Function/1
  Subtract2/1 -> Gbpn/1
  Qbp/1 -> Subsystem/1(QbpIC)
  Subsystem/1(Qbp) -> Divide/2
  Gsleep/1 -> Divide3/2, Divide2/1
  Divide3/1 -> GbO2/1

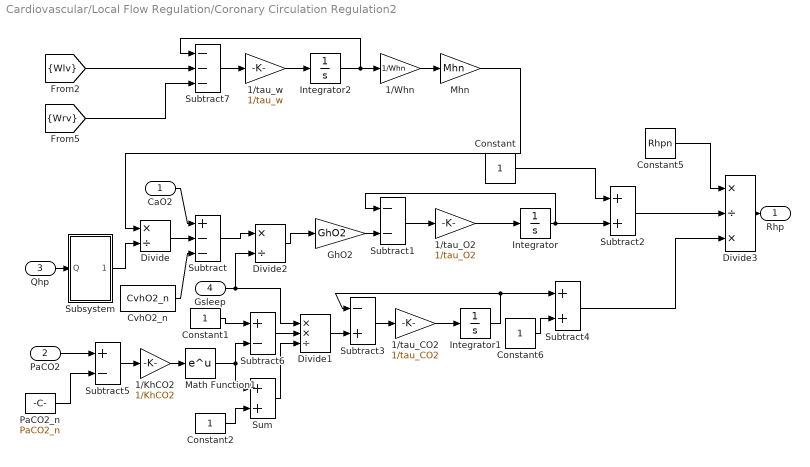
== system Cardiovascular/Local Flow Regulation/Coronary Circulation Regulation2 ==
  CaO2 : Inport
  PaCO2 : Inport  Port=2
  Qhp : Inport  Port=3
  Gsleep : Inport  Port=4
  1/KhCO2 : Gain  Gain=1/KhCO2
  1/Whn : Gain  Gain=1/Whn
  1/tau_CO2 : Gain  Gain=1/tau_CO2
  1/tau_O2 : Gain  Gain=1/tau_O2
  1/tau_w : Gain  Gain=1/tau_w
  Constant{,1..2,6} (4 alike) : Constant  Value=1  OutDataType=sfix(16)  ConRadixGroup=Use specified scaling  OutScaling=2^0  SampleTime=inf  FramePeriod=inf
  Constant5 : Constant  Value=Rhpn  OutDataType=sfix(16)  ConRadixGroup=Use specified scaling  OutScaling=2^0  SampleTime=inf  FramePeriod=inf
  CvhO2_n : Constant  Value=CvhO2_n  OutDataType=sfix(16)  ConRadixGroup=Use specified scaling  OutScaling=2^0  SampleTime=inf  FramePeriod=inf
  Divide : Product  Inputs=*/  OutScaling=2^-10
  Divide1 : Product  Inputs=**/  OutScaling=2^-10
  Divide2 : Product  Inputs=*/  OutScaling=2^-10
  Divide3 : Product  Inputs=*/*  OutScaling=2^-10
  GhO2 : Gain  Gain=GhO2
  Integrator : Integrator
  Integrator1 : Integrator
  Integrator2 : Integrator
  Math Function1 : Math  SaturateOnIntegerOverflow=on
  Mhn : Gain  Gain=Mhn
  PaCO2_n : Constant  Value=PaCO2_n  OutDataType=sfix(16)  ConRadixGroup=Use specified scaling  OutScaling=2^0  SampleTime=inf  FramePeriod=inf
  Subsystem : Subsystem
  Subtract : Sum  Inputs=+--  OutScaling=2^-10
  Subtract1 : Sum  Inputs=--  OutScaling=2^-10
  Subtract2 : Sum  OutScaling=2^-10
  Subtract3 : Sum  Inputs=-+  OutScaling=2^-10
  Subtract4 : Sum  OutScaling=2^-10
  Subtract5 : Sum  Inputs=+-  OutScaling=2^-10
  Subtract6 : Sum  Inputs=+-  OutScaling=2^-10
  Subtract7 : Sum  Inputs=---  OutScaling=2^-10
  Sum : Sum
  Rhp : Outport
  wires:
  Divide/1 -> Subtract/2
  CvhO2_n/1 -> Subtract/3
  GhO2/1 -> Subtract1/2
  Subtract1/1 -> 1/tau_O2/1
  1/tau_O2/1 -> Integrator/1
  Integrator/1 -> Subtract1/1, Subtract2/2
  Constant/1 -> Subtract2/1
  1/tau_CO2/1 -> Integrator1/1
  Integrator1/1 -> Subtract3/1, Subtract4/1
  Subtract3/1 -> 1/tau_CO2/1
  Subtract5/1 -> 1/KhCO2/1
  1/KhCO2/1 -> Math Function1/1
  Math Function1/1 -> Subtract6/2, Sum/1
  Constant2/1 -> Sum/2
  Subtract6/1 -> Divide1/2
  Sum/1 -> Divide1/3
  Constant5/1 -> Divide3/1
  Subtract2/1 -> Divide3/2
  Divide3/1 -> Rhp/1
  CaO2/1 -> Subtract/1
  PaCO2/1 -> Subtract5/1
  Constant6/1 -> Subtract4/2
  Subtract4/1 -> Divide3/3
  PaCO2_n/1 -> Subtract5/2
  Constant1/1 -> Subtract6/1
  Divide1/1 -> Subtract3/2
  1/tau_w/1 -> Integrator2/1
  Subtract7/1 -> 1/tau_w/1
  Integrator2/1 -> 1/Whn/1, Subtract7/1
  1/Whn/1 -> Mhn/1
  [Wlv] -> Subtract7/2
  [Wrv] -> Subtract7/3
  Subsystem/1(Qhp) -> Divide/2
  Qhp/1 -> Subsystem/1(Q)
  Mhn/1 -> Divide/1
  Gsleep/1 -> Divide2/2, Divide1/1
  Subtract/1 -> Divide2/1
  Divide2/1 -> GhO2/1

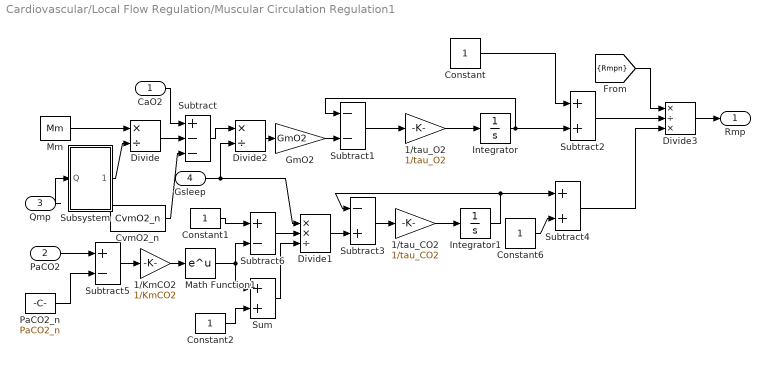
== system Cardiovascular/Local Flow Regulation/Muscular Circulation Regulation1 ==
  CaO2 : Inport
  PaCO2 : Inport  Port=2
  Qmp : Inport  Port=3
  Gsleep : Inport  Port=4
  1/KmCO2 : Gain  Gain=1/KmCO2
  1/tau_CO2 : Gain  Gain=1/tau_CO2
  1/tau_O2 : Gain  Gain=1/tau_O2
  Constant{,1..2,6} (4 alike) : Constant  Value=1  OutDataType=sfix(16)  ConRadixGroup=Use specified scaling  OutScaling=2^0  SampleTime=inf  FramePeriod=inf
  CvmO2_n : Constant  Value=CvmO2_n  OutDataType=sfix(16)  ConRadixGroup=Use specified scaling  OutScaling=2^0  SampleTime=inf  FramePeriod=inf
  Divide : Product  Inputs=*/  OutScaling=2^-10
  Divide1 : Product  Inputs=**/  OutScaling=2^-10
  Divide2 : Product  Inputs=*/  OutScaling=2^-10
  Divide3 : Product  Inputs=*/*  OutScaling=2^-10
  GmO2 : Gain  Gain=GmO2
  Integrator : Integrator  LimitOutput=on  UpperSaturationLimit=10000  LowerSaturationLimit=0
  Integrator1 : Integrator
  Math Function1 : Math  SaturateOnIntegerOverflow=on
  Mm : Constant  Value=Mm  OutDataType=sfix(16)  ConRadixGroup=Use specified scaling  OutScaling=2^0  SampleTime=inf  FramePeriod=inf
  PaCO2_n : Constant  Value=PaCO2_n  OutDataType=sfix(16)  ConRadixGroup=Use specified scaling  OutScaling=2^0  SampleTime=inf  FramePeriod=inf
  Subsystem : Subsystem
  Subtract : Sum  Inputs=+--  OutScaling=2^-10
  Subtract1 : Sum  Inputs=--  OutScaling=2^-10
  Subtract2 : Sum  OutScaling=2^-10
  Subtract3 : Sum  Inputs=-+  OutScaling=2^-10
  Subtract4 : Sum  OutScaling=2^-10
  Subtract5 : Sum  Inputs=+-  OutScaling=2^-10
  Subtract6 : Sum  Inputs=+-  OutScaling=2^-10
  Sum : Sum
  Rmp : Outport
  wires:
  Mm/1 -> Divide/1
  Divide/1 -> Subtract/2
  CvmO2_n/1 -> Subtract/3
  GmO2/1 -> Subtract1/2
  Subtract1/1 -> 1/tau_O2/1
  1/tau_O2/1 -> Integrator/1
  Integrator/1 -> Subtract1/1, Subtract2/2
  Constant/1 -> Subtract2/1
  1/tau_CO2/1 -> Integrator1/1
  Integrator1/1 -> Subtract3/1, Subtract4/1
  Subtract3/1 -> 1/tau_CO2/1
  Subtract5/1 -> 1/KmCO2/1
  1/KmCO2/1 -> Math Function1/1
  Math Function1/1 -> Subtract6/2, Sum/1
  Constant2/1 -> Sum/2
  Subtract6/1 -> Divide1/2
  Sum/1 -> Divide1/3
  [Rmpn] -> Divide3/1
  Subtract2/1 -> Divide3/2
  Divide3/1 -> Rmp/1
  CaO2/1 -> Subtract/1
  PaCO2/1 -> Subtract5/1
  Constant6/1 -> Subtract4/2
  Subtract4/1 -> Divide3/3
  PaCO2_n/1 -> Subtract5/2
  Constant1/1 -> Subtract6/1
  Divide1/1 -> Subtract3/2
  Qmp/1 -> Subsystem/1(Q)
  Subsystem/1(Qmp) -> Divide/2
  Subtract/1 -> Divide2/1
  Gsleep/1 -> Divide2/2, Divide1/1
  Divide2/1 -> GmO2/1

== system Cardiovascular/Pulmonary/SubSystem ==
  _ : Inport
  + : Inport  Port=2
  Saturation : Saturate  UpperLimit=10000  LowerLimit=0
  Sum : Sum  Inputs=|-+  SaturateOnIntegerOverflow=on  InputSameDT=on
  Out : Outport
  wires:
  _/1 -> Sum/1
  +/1 -> Sum/2
  Sum/1 -> Saturation/1
  Saturation/1 -> Out/1

== system Cardiovascular/Pulmonary/SubSystem1 ==
  _ : Inport
  + : Inport  Port=2
  Saturation : Saturate  UpperLimit=10000  LowerLimit=0
  Sum : Sum  Inputs=|-+  SaturateOnIntegerOverflow=on  InputSameDT=on
  Out : Outport
  wires:
  _/1 -> Sum/1
  +/1 -> Sum/2
  Sum/1 -> Saturation/1
  Saturation/1 -> Out/1

== system Cardiovascular/Pulmonary/SubSystem2 ==
  _ : Inport
  + : Inport  Port=2
  Saturation : Saturate  UpperLimit=10000  LowerLimit=0
  Sum : Sum  Inputs=|-+  SaturateOnIntegerOverflow=on  InputSameDT=on
  Out : Outport
  wires:
  Saturation/1 -> Out/1
  Sum/1 -> Saturation/1
  +/1 -> Sum/2
  _/1 -> Sum/1

== system Cardiovascular/Right Heart/Pmaxrv--Ppa ---------------------- Rrv ==
  Pmax : Inport
  P : Inport  Port=2
  Gain : Gain  Gain=KRrv  SaturateOnIntegerOverflow=on
  Product : Product  Inputs=/*  SaturateOnIntegerOverflow=on  RndMeth=Zero  InputSameDT=on
  Saturation : Saturate  UpperLimit=inf  LowerLimit=0.01
  Flow : Outport
  wires:
  Pmax/1 -> Gain/1
  Gain/1 -> Saturation/1
  P/1 -> Product/2
  Saturation/1 -> Product/1
  Product/1 -> Flow/1

== system Cardiovascular/Right Heart/SubSystem ==
  _ : Inport
  + : Inport  Port=2
  Saturation : Saturate  UpperLimit=10000  LowerLimit=0
  Sum : Sum  Inputs=|-+  SaturateOnIntegerOverflow=on  InputSameDT=on
  Out : Outport
  wires:
  _/1 -> Sum/1
  +/1 -> Sum/2
  Sum/1 -> Saturation/1
  Saturation/1 -> Out/1

== system Cardiovascular/Right Heart/SubSystem1 ==
  _ : Inport
  + : Inport  Port=2
  Saturation : Saturate  UpperLimit=10000  LowerLimit=0
  Sum : Sum  Inputs=|-+  SaturateOnIntegerOverflow=on  InputSameDT=on
  Out : Outport
  wires:
  Saturation/1 -> Out/1
  Sum/1 -> Saturation/1
  +/1 -> Sum/2
  _/1 -> Sum/1

== system Cardiovascular/SA-node and Autonomic Control/Heart Emaxlv ==
  ftbs : Inport
  Gbs(SI) : Inport  Port=2
  Basal_Emaxlv : Constant  Value=2.392  OutDataType=sfix(16)  ConRadixGroup=Use specified scaling  OutScaling=2^0  SampleTime=inf  FramePeriod=inf
  Constant : Constant  Value=ftbs_min  OutDataType=sfix(16)  ConRadixGroup=Use specified scaling  OutScaling=2^0  SampleTime=inf  FramePeriod=inf
  Gain_Emaxlv : Gain  Gain=0.475  SaturateOnIntegerOverflow=on
  Math Function : Math  Operator=log  SaturateOnIntegerOverflow=on
  Product3 : Product  SaturateOnIntegerOverflow=on  InputSameDT=on
  Saturation : Saturate  UpperLimit=inf  LowerLimit=1
  Sum : Sum  Inputs=+-  SaturateOnIntegerOverflow=on  InputSameDT=on
  Sum1 : Sum  SaturateOnIntegerOverflow=on  InputSameDT=on
  Transfer Fcn : TransferFcn  Denominator=[toux(1) 1]
  Transport Delay : TransportDelay  DelayTime=Dx(1)  BufferSize=19456
  Emaxlv : Outport
  wires:
  ftbs/1 -> Transport Delay/1
  Transport Delay/1 -> Sum/1
  Constant/1 -> Sum/2
  Sum/1 -> Saturation/1
  Saturation/1 -> Math Function/1
  Math Function/1 -> Gain_Emaxlv/1
  Transfer Fcn/1 -> Sum1/1
  Sum1/1 -> Emaxlv/1
  Basal_Emaxlv/1 -> Sum1/2
  Gbs(SI)/1 -> Product3/2
  Gain_Emaxlv/1 -> Product3/1
  Product3/1 -> Transfer Fcn/1

== system Cardiovascular/SA-node and Autonomic Control/Heart Emaxrv ==
  ftbs : Inport
  Gbs(SI) : Inport  Port=2
  Constant : Constant  Value=ftbs_min  OutDataType=sfix(16)  ConRadixGroup=Use specified scaling  OutScaling=2^0  SampleTime=inf  FramePeriod=inf
  Constant1 : Constant  Value=initx(2)  OutDataType=sfix(16)  ConRadixGroup=Use specified scaling  OutScaling=2^0  SampleTime=inf  FramePeriod=inf
  Gain_Emaxrv : Gain  Gain=0.282  SaturateOnIntegerOverflow=on
  Math Function : Math  Operator=log  SaturateOnIntegerOverflow=on
  Product3 : Product  SaturateOnIntegerOverflow=on  InputSameDT=on
  Saturation : Saturate  UpperLimit=inf  LowerLimit=1
  Sum : Sum  Inputs=|+-  SaturateOnIntegerOverflow=on  InputSameDT=on
  Sum1 : Sum  SaturateOnIntegerOverflow=on  InputSameDT=on
  Transfer Fcn : TransferFcn  Denominator=[toux(2) 1]
  Transport Delay : TransportDelay  DelayTime=Dx(2)  BufferSize=19456
  Emaxrv : Outport
  wires:
  Constant1/1 -> Sum1/2
  Sum1/1 -> Emaxrv/1
  Transfer Fcn/1 -> Sum1/1
  Math Function/1 -> Gain_Emaxrv/1
  Saturation/1 -> Math Function/1
  Sum/1 -> Saturation/1
  Constant/1 -> Sum/2
  Transport Delay/1 -> Sum/1
  ftbs/1 -> Transport Delay/1
  Gbs(SI)/1 -> Product3/2
  Gain_Emaxrv/1 -> Product3/1
  Product3/1 -> Transfer Fcn/1

== system Cardiovascular/SA-node and Autonomic Control/Left Ventricle ==
  phi : Inport  Orientation=left
  Constant13 : Constant  Orientation=left  Value=Vulv  OutDataType=sfix(16)  ConRadixGroup=Use specified scaling  OutScaling=2^0  SampleTime=inf  FramePeriod=inf
  Constant14 : Constant  Orientation=left  Value=P0lv  OutDataType=sfix(16)  ConRadixGroup=Use specified scaling  OutScaling=2^0  SampleTime=inf  FramePeriod=inf
  Constant6 : Constant  Orientation=left  Value=1  OutDataType=sfix(16)  ConRadixGroup=Use specified scaling  OutScaling=2^0  SampleTime=inf  FramePeriod=inf
  Fcn : Fcn  Orientation=left  Expr=exp(u*KElv)-1
  Product4 : Product  Orientation=left  Inputs=3  SaturateOnIntegerOverflow=on  RndMeth=Zero  InputSameDT=on
  Product5 : Product  Orientation=left  Inputs=3  SaturateOnIntegerOverflow=on  RndMeth=Zero  InputSameDT=on
  SubSystem1 : Subsystem  Orientation=left
  Sum2 : Sum  Orientation=left  SaturateOnIntegerOverflow=on  InputSameDT=on
  Sum3 : Sum  Orientation=left  Inputs=-+  SaturateOnIntegerOverflow=on  InputSameDT=on
  Pmaxlv : Outport  Orientation=left
  wires:
  Sum2/1 -> Pmaxlv/1
  Product4/1 -> Sum2/1
  Product5/1 -> Sum2/2
  Fcn/1 -> Product5/1
  Constant14/1 -> Product5/2
  Sum3/1 -> Product5/3
  Constant6/1 -> Sum3/2
  Constant13/1 -> SubSystem1/1(_)
  [Vlv] -> SubSystem1/2(+)
  SubSystem1/1(Out) -> Product4/2
  phi/1 -> Sum3/1, Product4/3
  [Emaxlv] -> Product4/1
  [Vlv] -> Fcn/1

== system Cardiovascular/SA-node and Autonomic Control/RR Interval ==
  HP_SAnode : Inport
  Abs : Abs  SaturateOnIntegerOverflow=on  SampleTime=-1
  Derivative1 : Derivative
  If : If  IfExpression=u1 <0  ShowElse=off
  If Action Subsystem : Subsystem  TreatAsAtomicUnit=on
  Integrator : Integrator  ExternalReset=rising  UpperSaturationLimit=10  LowerSaturationLimit=0
  Integrator1 : Integrator  ExternalReset=rising  UpperSaturationLimit=10  LowerSaturationLimit=0
  Math Function : Math  Operator=reciprocal  SaturateOnIntegerOverflow=on
  Memory : Memory  Orientation=left
  Mux : Mux
  Saving varHeartPeriod : Subsystem
  Sign1 : Signum  ZeroCross=off
  Sum : Sum  Inputs=+-  SaturateOnIntegerOverflow=on
  Threshold Integrated HP : Constant  Value=1  OutDataType=sfix(16)  ConRadixGroup=Use specified scaling  OutScaling=2^0  SampleTime=inf  FramePeriod=inf
  Time Constant : Constant  Value=1  OutDataType=sfix(16)  ConRadixGroup=Use specified scaling  OutScaling=2^0  SampleTime=inf  FramePeriod=inf
  Heart_Period : Outport
  wires:
  Threshold Integrated HP/1 -> Sum/1
  Integrator/1 -> Sum/2
  Sum/1 -> If/1, Mux/2  "HPin"
  Memory/1 -> Integrator/2, Integrator1/2
  Sign1/1 -> Abs/1
  Derivative1/1 -> Sign1/1
  Abs/1 -> Memory/1  "Enable signal"
  HP_SAnode/1 -> Math Function/1
  Time Constant/1 -> Integrator1/1
  Integrator1/1 -> If Action Subsystem/1(In1), Mux/3  "HPout"
  If Action Subsystem/1(Out1) -> Derivative1/1, Heart_Period/1, Mux/4  "Heart Period"
  If/1 -> If Action Subsystem/Action
  Math Function/1 -> Integrator/1, Mux/1
  Mux/1 -> Saving varHeartPeriod/1(In1)

== system Cardiovascular/SA-node and Autonomic Control/Right Ventricle ==
  phi : Inport  Orientation=left
  Constant13 : Constant  Orientation=left  Value=Vurv  OutDataType=sfix(16)  ConRadixGroup=Use specified scaling  OutScaling=2^0  SampleTime=inf  FramePeriod=inf
  Constant14 : Constant  Orientation=left  Value=P0rv  OutDataType=sfix(16)  ConRadixGroup=Use specified scaling  OutScaling=2^0  SampleTime=inf  FramePeriod=inf
  Constant6 : Constant  Orientation=left  Value=1  OutDataType=sfix(16)  ConRadixGroup=Use specified scaling  OutScaling=2^0  SampleTime=inf  FramePeriod=inf
  Fcn : Fcn  Orientation=left  Expr=exp(u*KErv)-1
  Product4 : Product  Orientation=left  Inputs=3  SaturateOnIntegerOverflow=on  RndMeth=Zero  InputSameDT=on
  Product5 : Product  Orientation=left  Inputs=3  SaturateOnIntegerOverflow=on  RndMeth=Zero  InputSameDT=on
  SubSystem1 : Subsystem  Orientation=left
  Sum2 : Sum  Orientation=left  SaturateOnIntegerOverflow=on  InputSameDT=on
  Sum3 : Sum  Orientation=left  Inputs=-+  SaturateOnIntegerOverflow=on  InputSameDT=on
  Pmaxrv : Outport  Orientation=left
  wires:
  Constant6/1 -> Sum3/2
  Sum3/1 -> Product5/3
  Constant14/1 -> Product5/2
  Fcn/1 -> Product5/1
  Product5/1 -> Sum2/2
  Product4/1 -> Sum2/1
  Sum2/1 -> Pmaxrv/1
  [Emaxrv] -> Product4/1
  [Vrv] -> SubSystem1/2(+)
  Constant13/1 -> SubSystem1/1(_)
  SubSystem1/1(Out) -> Product4/2
  phi/1 -> Sum3/1, Product4/3
  [Vrv] -> Fcn/1

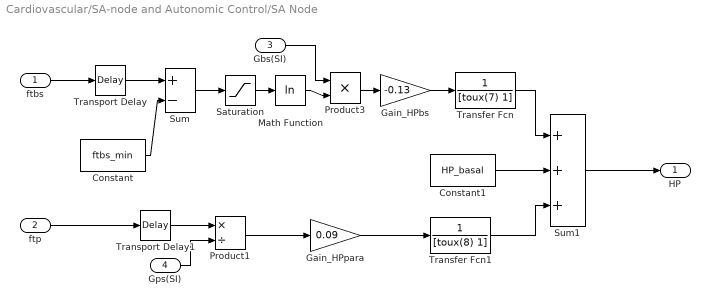
== system Cardiovascular/SA-node and Autonomic Control/SA Node ==
  ftbs : Inport
  ftp : Inport  Port=2
  Gbs(SI) : Inport  Port=3
  Gps(SI) : Inport  Port=4
  Constant : Constant  Value=ftbs_min  OutDataType=sfix(16)  ConRadixGroup=Use specified scaling  OutScaling=2^0  SampleTime=inf  FramePeriod=inf
  Constant1 : Constant  Value=HP_basal  OutDataType=sfix(16)  ConRadixGroup=Use specified scaling  OutScaling=2^0  SampleTime=inf  FramePeriod=inf
  Gain_HPbs : Gain  Gain=-0.13  SaturateOnIntegerOverflow=on
  Gain_HPpara : Gain  Gain=0.09  SaturateOnIntegerOverflow=on
  Math Function : Math  Operator=log  SaturateOnIntegerOverflow=on
  Product1 : Product  Inputs=*/  SaturateOnIntegerOverflow=on  InputSameDT=on
  Product3 : Product  SaturateOnIntegerOverflow=on  InputSameDT=on
  Saturation : Saturate  UpperLimit=inf  LowerLimit=1
  Sum : Sum  Inputs=+-  SaturateOnIntegerOverflow=on  InputSameDT=on
  Sum1 : Sum  Inputs=+++  SaturateOnIntegerOverflow=on  InputSameDT=on
  Transfer Fcn : TransferFcn  Denominator=[toux(7) 1]
  Transfer Fcn1 : TransferFcn  Denominator=[toux(8) 1]
  Transport Delay : TransportDelay  DelayTime=Dx(7)  BufferSize=19456
  Transport Delay1 : TransportDelay  DelayTime=Dx(8)  BufferSize=18432
  HP : Outport
  wires:
  ftbs/1 -> Transport Delay/1
  Transport Delay/1 -> Sum/1
  Constant/1 -> Sum/2
  Sum/1 -> Saturation/1
  Saturation/1 -> Math Function/1
  Math Function/1 -> Product3/2
  Gain_HPbs/1 -> Transfer Fcn/1
  Transfer Fcn/1 -> Sum1/1
  Sum1/1 -> HP/1
  Constant1/1 -> Sum1/2
  ftp/1 -> Transport Delay1/1
  Transport Delay1/1 -> Product1/1
  Gain_HPpara/1 -> Transfer Fcn1/1
  Transfer Fcn1/1 -> Sum1/3
  Gbs(SI)/1 -> Product3/1
  Product3/1 -> Gain_HPbs/1
  Product1/1 -> Gain_HPpara/1
  Gps(SI)/1 -> Product1/2

== system Cardiovascular/SA-node and Autonomic Control/phi ==
  HP : Inport
  Constant3 : Constant  Orientation=left  Value=0  OutDataType=sfix(16)  ConRadixGroup=Use specified scaling  OutScaling=2^0  SampleTime=inf  FramePeriod=inf
  Constant4 : Constant  Value=ksys  OutDataType=sfix(16)  ConRadixGroup=Use specified scaling  OutScaling=2^0  SampleTime=inf  FramePeriod=inf
  Constant5 : Constant  Value=Tsys0  OutDataType=sfix(16)  ConRadixGroup=Use specified scaling  OutScaling=2^0  SampleTime=inf  FramePeriod=inf
  Constant6 : Constant  Value=1  OutDataType=sfix(16)  ConRadixGroup=Use specified scaling  OutScaling=2^0  SampleTime=inf  FramePeriod=inf
  Data Store Memory : DataStoreMemory  DataStoreName=A  InitialValue=0
  Data Store Read : DataStoreRead  DataStoreName=A  SampleTime=0
  Fcn1 : Fcn  Expr=sin(pi*u)^2
  Integrator : Integrator
  Math Function2 : Math  Operator=rem  SaturateOnIntegerOverflow=on
  Math Function3 : Math  Operator=reciprocal  SaturateOnIntegerOverflow=on
  Product : Product  SaturateOnIntegerOverflow=on  RndMeth=Zero  InputSameDT=on
  Product2 : Product  Inputs=/*  SaturateOnIntegerOverflow=on  RndMeth=Zero  InputSameDT=on
  Product3 : Product  Inputs=*/  SaturateOnIntegerOverflow=on  RndMeth=Zero  InputSameDT=on
  SubSystem : Subsystem  TreatAsAtomicUnit=on
  Sum1 : Sum  Inputs=-+  SaturateOnIntegerOverflow=on  InputSameDT=on
  Switch : Switch  Threshold=1  SaturateOnIntegerOverflow=on  InputSameDT=on
  phi : Outport
  wires:
  Product3/1 -> Product/2
  Sum1/1 -> Product3/2
  Constant5/1 -> Sum1/2
  Product2/1 -> Sum1/1
  Constant4/1 -> Product2/2
  Constant3/1 -> Switch/1
  Product/1 -> Switch/2, Switch/3
  Fcn1/1 -> phi/1
  HP/1 -> SubSystem/1(In1)  "heart period"
  Switch/1 -> Fcn1/1, SubSystem/Trigger
  Data Store Read/1 -> Product3/1, Product2/1, Math Function3/1  "heart period"
  Constant6/1 -> Math Function2/2
  Math Function2/1 -> Product/1  "u"
  Math Function3/1 -> Integrator/1
  Integrator/1 -> Math Function2/1
